simulink model "two_mass_oscillator"  (R2022b)
settings: Solver=FixedStepAuto  StartTime=0.0  StopTime=180  FixedStep=0.001  RelTol=1e-3
model workspace (MAT data in the model file):
  Amplitude = 5
  J_1 = 1
  J_2 = 12
  d_1 = 1.5
  d_2 = 0
  k_1 = 10
  k_2 = 50
  omega = 3.1623
settings Model: Creator=yn05ehag  LastModifiedBy=oc47agip
settings SolverCC: AlgebraicLoopSolver=TrustRegion
settings DebuggingCC: UnconnectedInputMsg=warning  UnconnectedOutputMsg=warning  UnconnectedLineMsg=warning  SFMachineParentedDataDiag=warning
settings ModelReferenceCC: EnableRefExpFcnMdlSchedulingChecks=on
settings RTWCC: DLArmComputeVersion=19.05

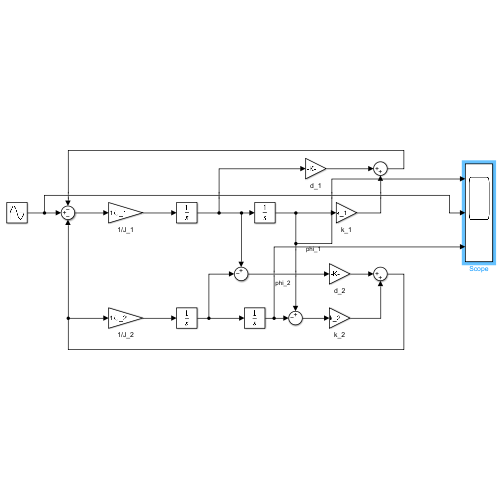
[thumbnail: Simulink's stored preview of the top-level diagram]
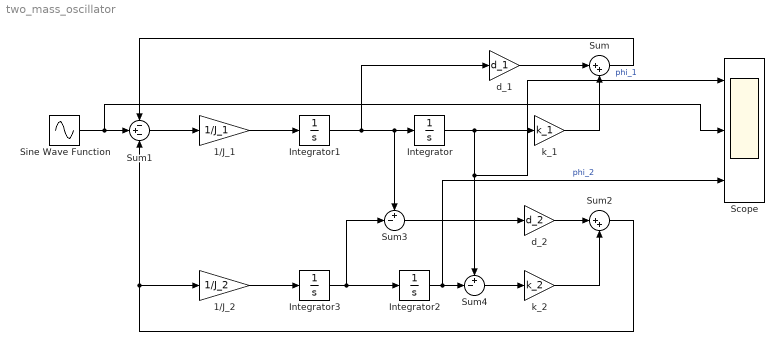
== system two_mass_oscillator ==
  1/J_1 : Gain  Gain=1/J_1
  1/J_2 : Gain  Gain=1/J_2
  Integrator{,1..3} (4 alike) : Integrator
  Scope : Scope  NumInputPorts=3
  Sine Wave Function : Sin  Amplitude=Amplitude  Frequency=omega  Phase=pi/2  SampleTime=0
  Sum : Sum  Inputs=|++
  Sum1 : Sum  Inputs=-+-
  Sum2 : Sum  Inputs=|++
  Sum3 : Sum  Inputs=+-|
  Sum4 : Sum  Inputs=+-|
  d_1 : Gain  Gain=d_1
  d_2 : Gain  Gain=d_2
  k_1 : Gain  Gain=k_1
  k_2 : Gain  Gain=k_2
  wires:
  Integrator1/1 -> Integrator/1, Sum3/1, d_1/1
  Integrator/1 -> Sum4/1, Scope/1, k_1/1  "phi_1"
  1/J_1/1 -> Integrator1/1
  d_1/1 -> Sum/1
  k_1/1 -> Sum/2
  Sine Wave Function/1 -> Sum1/2, Scope/2
  Sum/1 -> Sum1/1
  Sum1/1 -> 1/J_1/1
  k_2/1 -> Sum2/2
  d_2/1 -> Sum2/1
  Sum2/1 -> 1/J_2/1, Sum1/3
  Integrator3/1 -> Integrator2/1, Sum3/2
  1/J_2/1 -> Integrator3/1
  Sum3/1 -> d_2/1
  Integrator2/1 -> Scope/3, Sum4/2  "phi_2"
  Sum4/1 -> k_2/1
